simulink model "model_sinus_gust"  (R2020b)
settings: Solver=VariableStepAuto  StartTime=0.0  StopTime=10.0  RelTol=1e-3
undefined symbols (not defined in the file or in its folder): sinus_gust
settings Model: Creator=C:\Users\Dogukan  LastModifiedBy=C:\Users\Dogukan

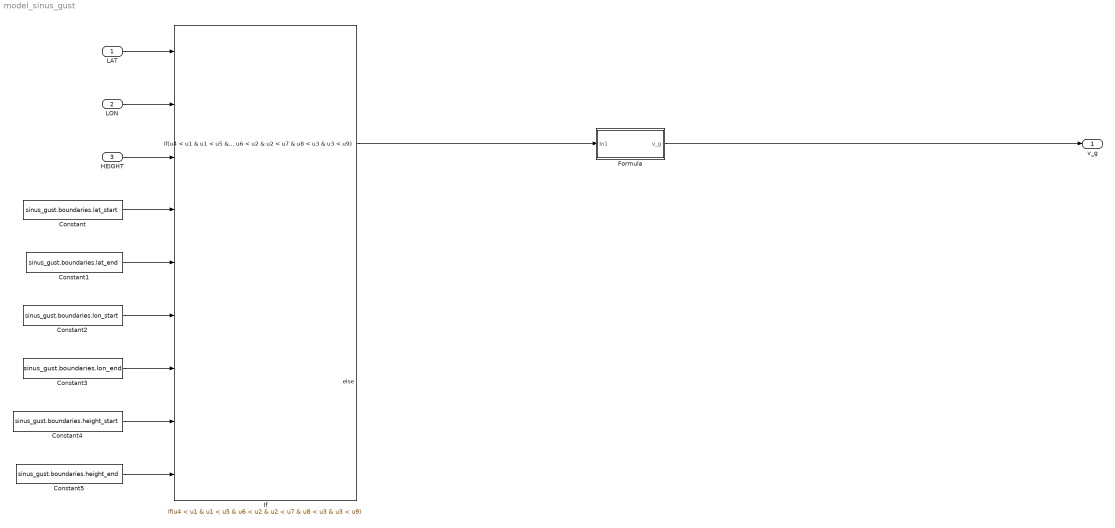
== system model_sinus_gust ==
  LAT : Inport
  LON : Inport  Port=2
  HEIGHT : Inport  Port=3
  Constant : Constant  Value=sinus_gust.boundaries.lat_start
  Constant1 : Constant  Value=sinus_gust.boundaries.lat_end
  Constant2 : Constant  Value=sinus_gust.boundaries.lon_start
  Constant3 : Constant  Value=sinus_gust.boundaries.lon_end
  Constant4 : Constant  Value=sinus_gust.boundaries.height_start
  Constant5 : Constant  Value=sinus_gust.boundaries.height_end
  Formula : Subsystem
  If : If  NumInputs=9  IfExpression=u4 < u1 & u1 < u5 & u6 < u2 & u2 < u7 & u8 < u3 & u3 < u9
  v_g : Outport
  wires:
  LON/1 -> If/2
  LAT/1 -> If/1
  HEIGHT/1 -> If/3
  Constant/1 -> If/4
  Constant1/1 -> If/5
  Constant2/1 -> If/6
  Constant3/1 -> If/7
  Constant4/1 -> If/8
  Constant5/1 -> If/9
  If/1 -> Formula/1(In1)
  Formula/1(v_g) -> v_g/1

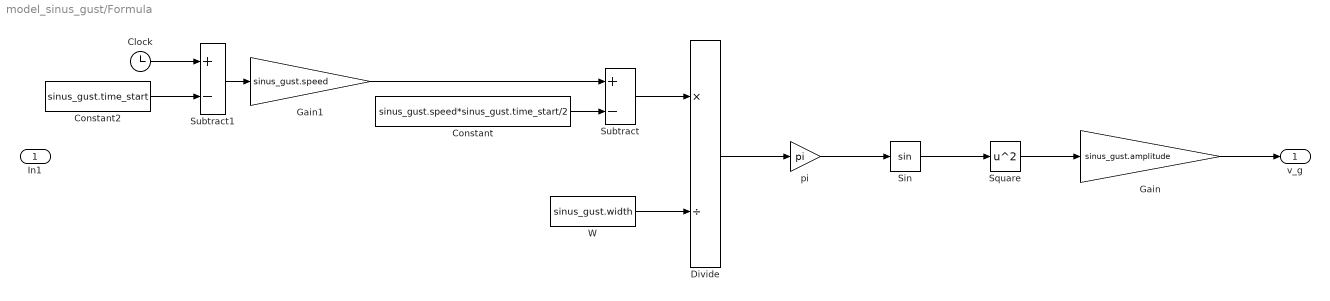
== system model_sinus_gust/Formula ==
  In1 : Inport
  Clock : Clock
  Constant : Constant  Value=sinus_gust.speed*sinus_gust.time_start/2
  Constant2 : Constant  Value=sinus_gust.time_start
  Divide : Product  Inputs=*/
  Gain : Gain  Gain=sinus_gust.amplitude
  Gain1 : Gain  Gain=sinus_gust.speed
  Sin : Trigonometry
  Square : Math  Operator=square  SaturateOnIntegerOverflow=on
  Subtract : Sum  Inputs=+-
  Subtract1 : Sum  Inputs=+-
  W : Constant  Value=sinus_gust.width
  pi : Gain  Gain=pi
  v_g : Outport
  wires:
  Gain/1 -> v_g/1
  Square/1 -> Gain/1
  Sin/1 -> Square/1
  pi/1 -> Sin/1
  W/1 -> Divide/2
  Divide/1 -> pi/1
  Constant/1 -> Subtract/2
  Subtract/1 -> Divide/1
  Clock/1 -> Subtract1/1
  Constant2/1 -> Subtract1/2
  Subtract1/1 -> Gain1/1
  Gain1/1 -> Subtract/1
